simulink model "TrafficLight"  (R2022b)
settings: Solver=VariableStepAuto  StartTime=0.0  StopTime=10.0  RelTol=1e-3
settings Model: Creator=ahmed  LastModifiedBy=ahmed

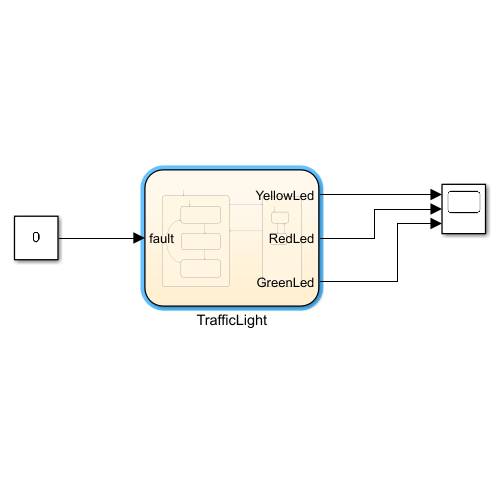
[thumbnail: Simulink's stored preview of the top-level diagram]
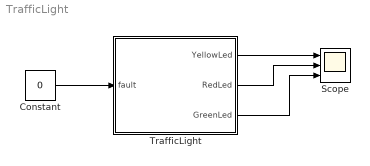
== system TrafficLight ==
  Constant : Constant  Value=0
  Scope : Scope  NumInputPorts=3
  TrafficLight : Stateflow chart  TreatAsAtomicUnit=on
  wires:
  TrafficLight/1(YellowLed) -> Scope/1
  TrafficLight/2(RedLed) -> Scope/2
  TrafficLight/3(GreenLed) -> Scope/3
  Constant/1 -> TrafficLight/1(fault)

== stateflow chart TrafficLight/TrafficLight ==
  state NormalMode
    state Stop
      en:
      RedLed = 1;
      ex:
      RedLed = 0;
    state Go
      en:
      GreenLed = 1;
      ex:
      GreenLed = 0;
    state PrepStop
      en:
      YellowLed = 1;
      ex:
      YellowLed = 0;
    (default) -> Stop
    PrepStop -> Stop : after(1,sec)
    Stop -> Go : after(1 ,sec)
    Go -> PrepStop : after(1,sec)
  state FaultMode
    state LedOn
      en:
      RedLed = 1;
    state LedOff
      en:
      RedLed = 0;
    (default) -> LedOn
    LedOn -> LedOff : after(1,sec)
    LedOff -> LedOn : after(1,sec)
  (default) -> NormalMode
  NormalMode -> FaultMode : [fault == 1]
  FaultMode -> NormalMode : [fault == 0]
  data: fault input; YellowLed output; RedLed output; GreenLed output
